simulink model "problem3"  (R2020b)
settings: Solver=VariableStepAuto  StartTime=0.0  StopTime=10.0  RelTol=1e-3
PreLoadFcn:
  | init
values from neighbouring files (symbols this model uses):
  ctrl = 0    [init.m]
  g = 32.18    [init.m]
  I = 5    [init.m]
  Kf = 1    [init.m]
  m = 50    [init.m]
  mu = [0 .4 .8 .97 1.0 .98 .96 .94 .92 .9 .88 .855 .83 .81 .79 .77 .75 .73 .72 .71 .7]    [init.m]
  PBmax = 1500    [init.m]
  Rr = 15/12    (= 1.25)    [init.m]
  slip = (0:.05:1.0)    [init.m]
  TB = 0.01    [init.m]
  v0 = 88    [init.m]
undefined symbols (not defined in the file or in its folder): sigbuilder_block
settings Model: Creator=ARPITA  LastModifiedBy=ARPITA

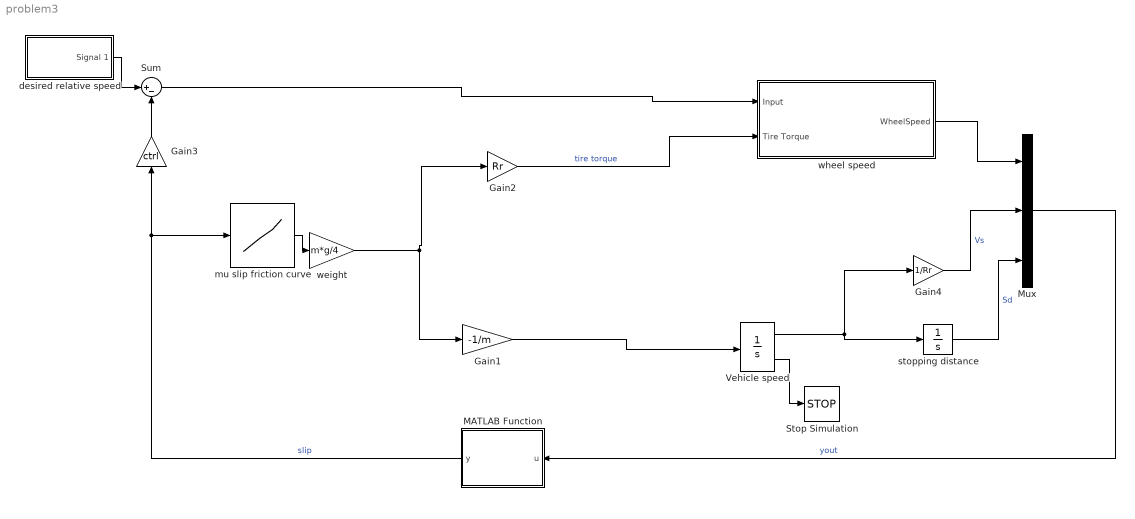
== system problem3 ==
  Gain1 : Gain  Gain=-1/m
  Gain2 : Gain  Gain=Rr
  Gain3 : Gain  Gain=ctrl
  Gain4 : Gain  Gain=1/Rr
  MATLAB Function : MATLAB Function  TreatAsAtomicUnit=on
  Mux : Mux  Inputs=3
  Stop Simulation : Stop
  Sum : Sum  Inputs=|+-
  Vehicle speed : Integrator  InitialCondition=v0  LimitOutput=on  UpperSaturationLimit=1000  LowerSaturationLimit=0  ShowSaturationPort=on
  desired relative speed : Subsystem  Tag=STV Subsys  LoadFcn=sigbuilder_block('load');  StartFcn=sigbuilder_block('start');  StopFcn=sigbuilder_block('stop');  ClipboardFcn=sigbuilder_block('clipboard');  mask(Sigbuilder block){tuvar=[0:10]}
      mask help: Simulink:masks:SigbuilderBlock_MD
      mask init:
      | if ~strcmp(get_param(bdroot(gcbh),'SimulationStatus'),'stopped') tuvar = sigbuilder_block('maskInit'); end
      settings: CopyFcn=sigbuilder_block('copy');  DeleteFcn=sigbuilder_block('delete');  ModelCloseFcn=sigbuilder_block('modelClose');  PreSaveFcn=sigbuilder_block('preSave');  PauseFcn=sigbuilder_block('pause');  ContinueFcn=sigbuilder_block('continue');  NameChangeFcn=sigbuilder_block('namechange');  OpenFcn=sigbuilder_block('open',[437.6 153 550.4 359.25 ]);  CloseFcn=sigbuilder_block('close');
      mask Display: plot(0, 0, 100, 100,[2, 2, 32, 32, 2], [68, 8, 8, 68, 68],[32, 2], [38, 38], [32, 19, 2],[53, 60, 44], [32, 17, 17, 2],[16, 16, 31, 31]);txt = getActiveGroup(gcbh);text(2, 100, txt,'verticalAlignment', 'top');
  mu slip friction curve : Lookup_n-D  NumberOfTableDimensions=1  BreakpointsForDimension1=slip  Table=mu  InternalRulePriority=Speed  RndMeth=Simplest  InputSameDT=on
  stopping distance : Integrator
  weight : Gain  Gain=m*g/4
  wheel speed : Subsystem
  wires:
  desired relative speed/1(Signal 1) -> Sum/1
  Gain3/1 -> Sum/2
  mu slip friction curve/1 -> weight/1
  weight/1 -> Gain2/1, Gain1/1
  Gain1/1 -> Vehicle speed/1
  Vehicle speed/1 -> stopping distance/1, Gain4/1
  Vehicle speed/2 -> Stop Simulation/1
  Gain4/1 -> Mux/2  "Vs"
  stopping distance/1 -> Mux/3  "Sd"
  MATLAB Function/1(y) -> Gain3/1, mu slip friction curve/1  "slip"
  Mux/1 -> MATLAB Function/1(u)  "yout"
  Sum/1 -> wheel speed/1(Input)
  Gain2/1 -> wheel speed/2(Tire Torque)  "tire torque"
  wheel speed/1(WheelSpeed) -> Mux/1

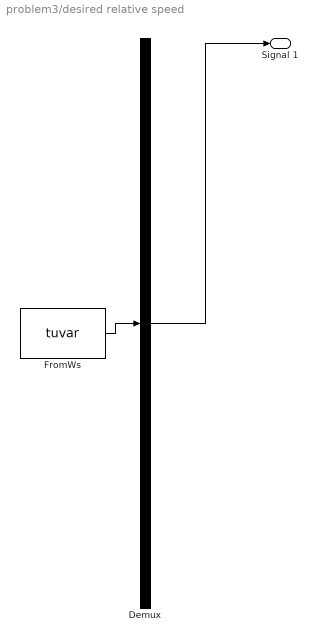
== system problem3/desired relative speed ==
  Demux : Demux  Tag=STV Demux  Outputs=1
      settings: DisplayOption=none
  FromWs : FromWorkspace  Tag=STV FromWs  VariableName=tuvar
      SigBuilderData=|
      | common.afterFinalStr = 'Extrapolate'
      | common.sampleTime = 0
      | dataSet.timeRange = [0 10]
      | dataSet.name = 'Group 1'
      | sbobj.Groups.Name = 'Group 1'
      | sbobj.Groups.Signals.Name = 'Signal 1'
      | sbobj.Groups.Signals.XData = [0 4 6 10]
      | sbobj.Groups.Signals.YData = [0.2 0.2 0.2 0.2]
  Signal 1 : Outport  Tag=STV Outport
  wires:
  Demux/1 -> Signal 1/1
  FromWs/1 -> Demux/1

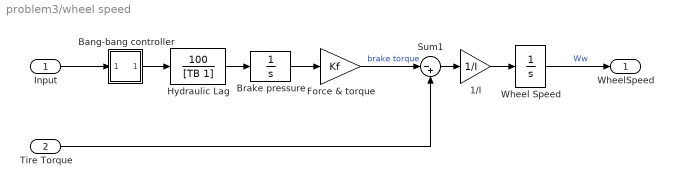
== system problem3/wheel speed ==
  Input : Inport  SampleTime=0
  Tire Torque : Inport  Port=2
  1/I : Gain  Gain=1/I  SaturateOnIntegerOverflow=on  OutDataTypeStr=Inherit: Same as input  ParamDataTypeStr=Inherit: Same as input
  Bang-bang controller : Subsystem  mask(Sign){}
      mask help: y = sign(x)
      mask Help: Sign Function:\n\t\t\ty = 1 if x > 0\n\t\t\ty = 0 if x = 0\n\t\t\ty = -1 if x < 0
      mask Display: plot(-50,-50,50,50,[-50,50],[0,0],[0,0],[-50,50],[-40,0],[-30,-30],[0,40],[30,30])
  Brake pressure : Integrator  LimitOutput=on  UpperSaturationLimit=PBmax  LowerSaturationLimit=0
  Force & torque : Gain  Gain=Kf  SaturateOnIntegerOverflow=on  OutDataTypeStr=Inherit: Same as input  ParamDataTypeStr=Inherit: Same as input
  "Hydraulic Lag " : TransferFcn  Numerator=[100]  Denominator=[TB 1]
  Sum1 : Sum  Inputs=|-+  InputSameDT=on  SaturateOnIntegerOverflow=on  OutDataTypeStr=Inherit: Same as first input
  Wheel Speed : Integrator  InitialCondition=v0/Rr  LimitOutput=on  UpperSaturationLimit=1000  LowerSaturationLimit=0
  WheelSpeed : Outport  VectorParamsAs1DForOutWhenUnconnected=off
  wires:
  "Hydraulic Lag "/1 -> Brake pressure/1
  Bang-bang controller/1(out_1) -> "Hydraulic Lag "/1
  Tire Torque/1 -> Sum1/2
  Wheel Speed/1 -> WheelSpeed/1  "Ww"
  Sum1/1 -> 1/I/1
  Brake pressure/1 -> Force & torque/1
  Force & torque/1 -> Sum1/1  "brake torque"
  Input/1 -> Bang-bang controller/1(in_1)
  1/I/1 -> Wheel Speed/1

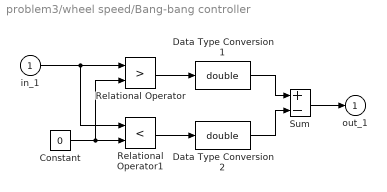
== system problem3/wheel speed/Bang-bang controller ==
  in_1 : Inport
  Constant : Constant  Value=0
  Data Type Conversion1 : DataTypeConversion  OutDataTypeStr=double  SaturateOnIntegerOverflow=on  RndMeth=Zero
  Data Type Conversion2 : DataTypeConversion  OutDataTypeStr=double  SaturateOnIntegerOverflow=on  RndMeth=Zero
  Relational Operator : RelationalOperator  Operator=>  OutDataTypeStr=boolean  RndMeth=Nearest  InputSameDT=on
  Relational Operator1 : RelationalOperator  Operator=<  OutDataTypeStr=boolean  RndMeth=Nearest  InputSameDT=on
  Sum : Sum  Inputs=+-  InputSameDT=on  SaturateOnIntegerOverflow=on  OutDataTypeStr=Inherit: Same as first input
  out_1 : Outport  InitialOutput=0  VectorParamsAs1DForOutWhenUnconnected=off
  wires:
  Data Type Conversion2/1 -> Sum/2
  Data Type Conversion1/1 -> Sum/1
  Sum/1 -> out_1/1
  Relational Operator/1 -> Data Type Conversion1/1
  Relational Operator1/1 -> Data Type Conversion2/1
  Constant/1 -> Relational Operator/2, Relational Operator1/2
  in_1/1 -> Relational Operator1/1, Relational Operator/1

== matlab function problem3/MATLAB Function ==
  data: u input; y output

function y = fcn(u)

y = 1.0 - u(1)/(u(2) + (u(2)==0)*eps);
